simulink model "Ejercicio_21_23_02_17"  (R2013a)
settings: Solver=ode45  StartTime=0.0  StopTime=10  RelTol=1e-3
settings Model: Creator=Miguel  LastModifiedBy=Miguel

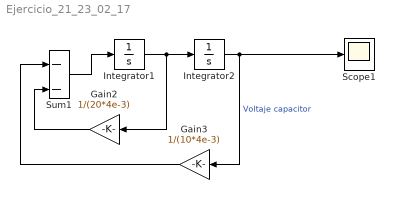
== system Ejercicio_21_23_02_17 ==
  Gain2 : Gain  Gain=1/(20*4e-3)
  Gain3 : Gain  Gain=1/(10*4e-3)
  Integrator1 : Integrator
  Integrator2 : Integrator  InitialCondition=2
  Scope1 : Scope
      settings: ShowLegends=on
  Sum1 : Sum  Inputs=|--
  wires:
  Integrator1/1 -> Gain2/1, Integrator2/1
  Sum1/1 -> Integrator1/1
  Integrator2/1 -> Scope1/1, Gain3/1  "Voltaje capacitor"
  Gain2/1 -> Sum1/2
  Gain3/1 -> Sum1/1
